simulink model "hdlFrame_HarrisCornerDetection_2D_NPSS"  (R2023a)
settings: Solver=FixedStepDiscrete  StartTime=0.0  StopTime=0  RelTol=1e-3
InitFcn:
  | slfeature('SLBlockSimThruCGXE', 2);
  | slfeature('SLCGEVCGDomainSubsystem', 1);
model workspace (MAT data in the model file):
  h = 5
  im = [0.16862745098 0.172549019608 0.16862745098 0.16862745098 0.172549019608 0.176470588235 0.16862745098 0.172549019608 0.172549019608 0.164705882353 0.160784313725 0.164705882353 ... (196608 elements, 384x512)]
  w = 5
undefined symbols (not defined in the file or in its folder): checkerboard, gray
(part 2 of 2)

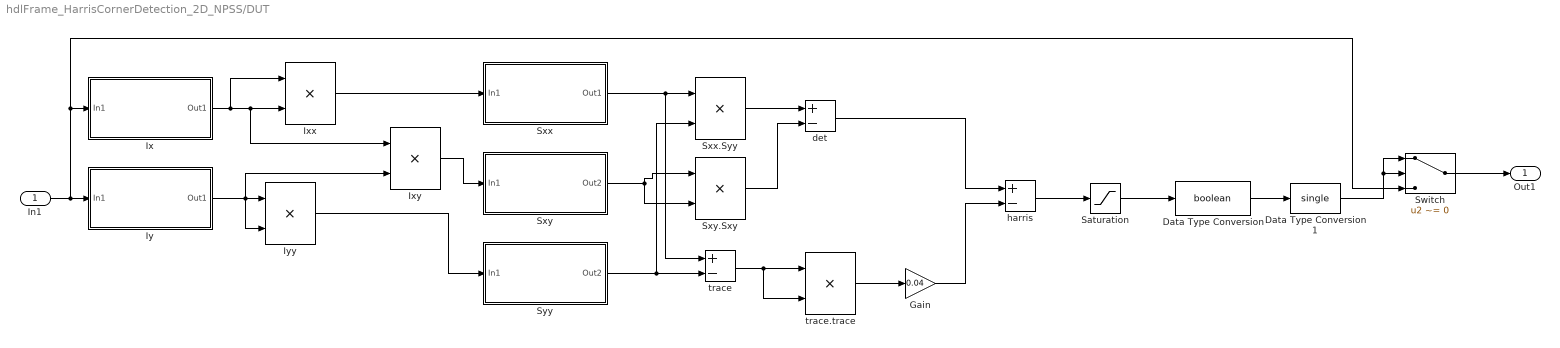
== system hdlFrame_HarrisCornerDetection_2D_NPSS/DUT ==
  In1 : Inport
  Data Type Conversion : DataTypeConversion  OutDataTypeStr=boolean  SaturateOnIntegerOverflow=off  RndMeth=Floor
  Data Type Conversion1 : DataTypeConversion  OutDataTypeStr=single  SaturateOnIntegerOverflow=off  RndMeth=Floor
  Gain : Gain  Gain=0.04
  Ix : Subsystem  TreatAsAtomicUnit=on
      settings: RTWSystemCode=Nonreusable function
  Ixx : Product
  Ixy : Product
  Iy : Subsystem  TreatAsAtomicUnit=on
      settings: RTWSystemCode=Nonreusable function
  Iyy : Product
  Saturation : Saturate  UpperLimit=1  LowerLimit=0
  Switch : Switch  Criteria=u2 ~= 0  SaturateOnIntegerOverflow=off  InputSameDT=off
  Sxx : Subsystem  TreatAsAtomicUnit=on
      settings: RTWSystemCode=Nonreusable function
  Sxx.Syy : Product
  Sxy : Subsystem  TreatAsAtomicUnit=on
      settings: RTWSystemCode=Nonreusable function
  Sxy.Sxy : Product
  Syy : Subsystem  TreatAsAtomicUnit=on
      settings: RTWSystemCode=Nonreusable function
  det : Sum  Inputs=+-
  harris : Sum  Inputs=+-
  trace : Sum  Inputs=+-
  trace.trace : Product
  Out1 : Outport
  wires:
  Ixy/1 -> Sxy/1(In1)
  Switch/1 -> Out1/1
  Sxy/1(Out2) -> Sxy.Sxy/1, Sxy.Sxy/2
  Iyy/1 -> Syy/1(In1)
  Syy/1(Out2) -> trace/2, Sxx.Syy/2
  Iy/1(Out1) -> Ixy/2, Iyy/1, Iyy/2
  Sxx/1(Out1) -> trace/1, Sxx.Syy/1
  Ix/1(Out1) -> Ixx/2, Ixy/1, Ixx/1
  Ixx/1 -> Sxx/1(In1)
  Sxx.Syy/1 -> det/1
  Sxy.Sxy/1 -> det/2
  trace/1 -> trace.trace/2, trace.trace/1
  trace.trace/1 -> Gain/1
  det/1 -> harris/1
  Gain/1 -> harris/2
  harris/1 -> Saturation/1
  In1/1 -> Switch/3, Ix/1(In1), Iy/1(In1)
  Data Type Conversion/1 -> Data Type Conversion1/1
  Data Type Conversion1/1 -> Switch/1, Switch/2
  Saturation/1 -> Data Type Conversion/1

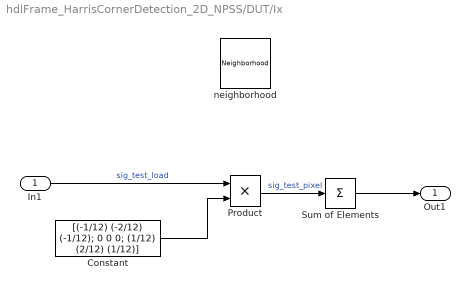
== system hdlFrame_HarrisCornerDetection_2D_NPSS/DUT/Ix ==
  In1 : Inport  PartitionDimension=[1 2]  PartitionWidth=[1 1]  PartitionOffset=[0 0]
  Constant : Constant  Value="[(-1/12) (-2/12)  (-1/12); 0 0 0; (1/12) (2/12) (1/12)]"  VectorParams1D=off  OutDataTypeStr=single
  Product : Product
  Sum of Elements : Sum  Inputs=+
  neighborhood : Neighborhood
  Out1 : Outport  ConcatenationDimension=[1 2]
  wires:
  Product/1 -> Sum of Elements/1  "sig_test_pixel"
  In1/1 -> Product/1  "sig_test_load"
  Constant/1 -> Product/2
  Sum of Elements/1 -> Out1/1

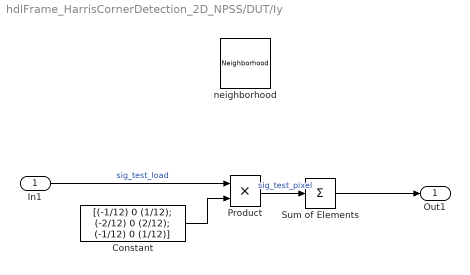
== system hdlFrame_HarrisCornerDetection_2D_NPSS/DUT/Iy ==
  In1 : Inport  PartitionDimension=[1 2]  PartitionWidth=[1 1]  PartitionOffset=[0 0]
  Constant : Constant  Value=[(-1/12) 0 (1/12); (-2/12) 0 (2/12); (-1/12) 0 (1/12)]  VectorParams1D=off  OutDataTypeStr=single
  Product : Product
  Sum of Elements : Sum  Inputs=+
  neighborhood : Neighborhood
  Out1 : Outport  ConcatenationDimension=[1 2]
  wires:
  Product/1 -> Sum of Elements/1  "sig_test_pixel"
  In1/1 -> Product/1  "sig_test_load"
  Constant/1 -> Product/2
  Sum of Elements/1 -> Out1/1

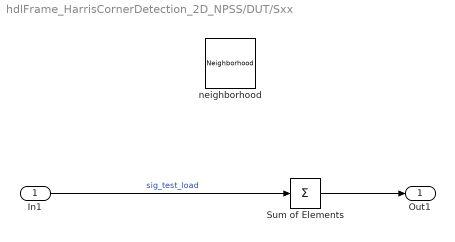
== system hdlFrame_HarrisCornerDetection_2D_NPSS/DUT/Sxx ==
  In1 : Inport  PartitionDimension=[1 2]  PartitionWidth=[1 1]  PartitionOffset=[0 0]
  Sum of Elements : Sum  Inputs=+
  neighborhood : Neighborhood
  Out1 : Outport  ConcatenationDimension=[1 2]
  wires:
  In1/1 -> Sum of Elements/1  "sig_test_load"
  Sum of Elements/1 -> Out1/1

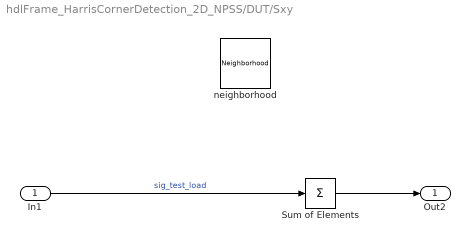
== system hdlFrame_HarrisCornerDetection_2D_NPSS/DUT/Sxy ==
  In1 : Inport  PartitionDimension=[1 2]  PartitionWidth=[1 1]  PartitionOffset=[0 0]
  Sum of Elements : Sum  Inputs=+
  neighborhood : Neighborhood
  Out2 : Outport  ConcatenationDimension=[1 2]
  wires:
  In1/1 -> Sum of Elements/1  "sig_test_load"
  Sum of Elements/1 -> Out2/1

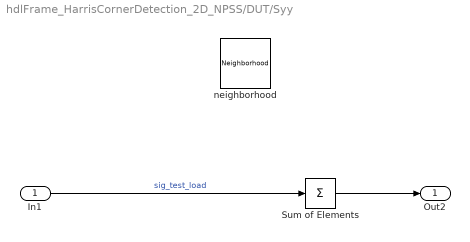
== system hdlFrame_HarrisCornerDetection_2D_NPSS/DUT/Syy ==
  In1 : Inport  PartitionDimension=[1 2]  PartitionWidth=[1 1]  PartitionOffset=[0 0]
  Sum of Elements : Sum  Inputs=+
  neighborhood : Neighborhood
  Out2 : Outport  ConcatenationDimension=[1 2]
  wires:
  In1/1 -> Sum of Elements/1  "sig_test_load"
  Sum of Elements/1 -> Out2/1
